simulink model "sim_model"  (Simulink 10.1)
settings: Solver=ode45  StartTime=0  StopTime=1  RelTol=0.001  EnableMultiTasking=on
libraries: fmu_me_lib x1
settings Model: Creator=Tin Rabuzin
settings DataIOCC: LimitDataPoints=on  OutputSaveName=simout  OutputOption=SpecifiedOutputTimes  OutputTimes=[0:0.1:1]
settings OptimizationCC: ExpressionDepthLimit=2147483647
settings DebuggingCC: SolverPrmCheckMsg=warning  FcnCallInpInsideContextMsg=warning  StateNameClashWarn=warning

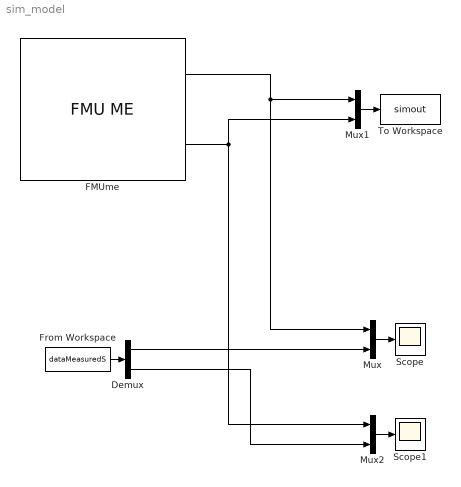
== system sim_model ==
  Demux : Demux  Outputs=2
  FMUme : fmu_me_lib/FMU ME  Description=Simulates an FMU for Model Exchange 1.0 or Model Exchange 2.0.  dummy=0
      settings: SourceProductName=The database C:\Users\meagh\AppData\Roaming\MathWorks\MATLAB\R2018b\slblocks_master.db is locked, or a table in the database is locked. (database is locked)
  From Workspace : FromWorkspace  VariableName=dataMeasuredS
  Mux : Mux  Inputs=2
  Mux1 : Mux  Inputs=2
  Mux2 : Mux  Inputs=2
  Scope : Scope
  Scope1 : Scope
  To Workspace : ToWorkspace  VariableName=simout  SaveFormat=Structure With Time  SampleTime=-1
  wires:
  Mux/1 -> Scope/1
  Mux1/1 -> To Workspace/1
  Mux2/1 -> Scope1/1
  Demux/2 -> Mux2/2
  From Workspace/1 -> Demux/1
  Demux/1 -> Mux/2
  FMUme/1 -> Mux/1, Mux1/1
  FMUme/2 -> Mux1/2, Mux2/1
